simulink model "B5b"  (Simulink 7.9)
settings: Solver=ode45  StartTime=0.0  StopTime=10.0  RelTol=1e-3
settings Model: Creator=Admin  LastModifiedBy=Admin

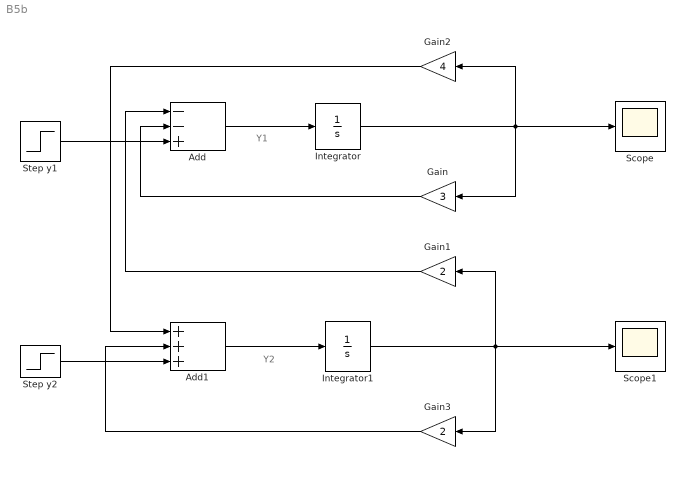
== system B5b ==
  note: Y1
  note: Y2
  Add : Sum  Inputs=--+
  Add1 : Sum  Inputs=+++
  Gain : Gain  Gain=3
  Gain1 : Gain  Gain=2
  Gain2 : Gain  Gain=4
  Gain3 : Gain  Gain=2
  Integrator : Integrator
  Integrator1 : Integrator
  Scope : Scope
  Scope1 : Scope
  Step y1 : Step  Time=0  Before=1  SampleTime=0
  Step y2 : Step  Time=0  Before=1  SampleTime=0
  wires:
  Add/1 -> Integrator/1
  Gain/1 -> Add/2
  Integrator/1 -> Scope/1, Gain/1, Gain2/1
  Integrator1/1 -> Scope1/1, Gain1/1, Gain3/1
  Gain1/1 -> Add/1
  Add1/1 -> Integrator1/1
  Gain2/1 -> Add1/1
  Gain3/1 -> Add1/2
  Step y1/1 -> Add/3
  Step y2/1 -> Add1/3
